simulink model "threeDiskOscillatorRig"  (R2024b)
settings: Solver=VariableStepAuto  StartTime=0.0  StopTime=simTime  RelTol=1e-8
values from neighbouring files (symbols this model uses):
  atan_scale = 100    [threeDiskOscillator.m]
  b_1 = mean(ECP_values([6 7]))    [threeDiskOscillator.m]
  b_2 = mean(ECP_values([8 9]))    [threeDiskOscillator.m]
  b_3 = mean(ECP_values([10 11]))    [threeDiskOscillator.m]
  B_change = [1 0;0 0]    [threeDiskOscillator.m]
  C = [  1 0 0 0 0 0 ... (first row only)    [threeDiskOscillator.m]
  C_aug = [C zeros(3,1)]    [threeDiskOscillator.m]
  C_D = C    [threeDiskOscillator.m]
  C_ref = pinv(C(3,:)/(eye(6) - F_d + G_d*K_c)*G_d*K_c)    [threeDiskOscillator.m]
  C_V_d = C_aug-P_V_d*C_f_aug    [threeDiskOscillator.m]
  F_aug = [F_d G_d(:,1);zeros(1,6) 1]    [threeDiskOscillator.m]
  F_D = F_d - G_f*M_d_va    [threeDiskOscillator.m]
  f_m = [0;0;0]    [threeDiskOscillator.m]
  f_m_time = 8.5    [threeDiskOscillator.m]
  f_u = [0;-0.1]    [threeDiskOscillator.m]
  f_u_time = 25    [threeDiskOscillator.m]
  F_V = F_a-L_V_d*C_f_aug    [threeDiskOscillator.m]
  G_aug = [G_d;0 0]    [threeDiskOscillator.m]
  G_D = G_d - G_f*N_D_d    [threeDiskOscillator.m]
  G_r1u2 = -(1/J_2)*G    [threeDiskOscillator.m]
  G_r1u2_d = c2d(G_r1u2,T_s, 'tustin')    [threeDiskOscillator.m]
  G_r1y1 = -(k_1/J_2)*G    [threeDiskOscillator.m]
  G_r1y1_d = c2d(G_r1y1,T_s, 'tustin')    [threeDiskOscillator.m]
  G_r1y2 = (s^2 + b_2/J_2*s + (k_1+k_2)/J_2)*G    [threeDiskOscillator.m]
  G_r1y2_d = c2d(G_r1y2,T_s, 'tustin')    [threeDiskOscillator.m]
  G_r1y3 = -(k_2/J_2)*G    [threeDiskOscillator.m]
  G_r1y3_d = c2d(G_r1y3,T_s, 'tustin')    [threeDiskOscillator.m]
  G_r2y2 = -(k_2/J_3)*G    [threeDiskOscillator.m]
  G_r2y2_d = c2d(G_r2y2,T_s, 'tustin')    [threeDiskOscillator.m]
  G_r2y3 = (s^2 + b_3/J_3*s + (k_2)/J_3)*G    [threeDiskOscillator.m]
  G_r2y3_d = c2d(G_r2y3,T_s, 'tustin')    [threeDiskOscillator.m]
  G_V = G_a    [threeDiskOscillator.m]
  h = double(vpasolve(eq_1,gg))    [threeDiskOscillator.m]
  J_1 = ECP_values(1)    [threeDiskOscillator.m]
  J_2 = ECP_values(2)    [threeDiskOscillator.m]
  J_3 = ECP_values(3)    [threeDiskOscillator.m]
  k_1 = ECP_values(4)    [threeDiskOscillator.m]
  k_2 = ECP_values(5)    [threeDiskOscillator.m]
  K_c = dlqr(F_d,G_d,Q_c,R_c)    [threeDiskOscillator.m]
  L_aug = dlqe(F_aug,eye(7),C_aug,1e-3*eye(7),sigma_meas(1,1).^2*eye(3))    [threeDiskOscillator.m]
  L_V_d = place(F_a',C_f_aug',vs_eig_d)'    [threeDiskOscillator.m]
  M_d_va = place(F_d,G_f,va_eig_d)    [threeDiskOscillator.m]
  mu_0 = -6.2064e-07    [threeDiskOscillator.m]
  N_D_d = pinv(G_f)*G_f    [threeDiskOscillator.m]
  P_V_d = C_aug*pinv(C_f_aug)    [threeDiskOscillator.m]
  sigma_meas = 0.0093*eye(3)    [threeDiskOscillator.m]
  sigma_r2 = 3.6238e-05    [threeDiskOscillator.m]
  T_Cm = ECP_values(13)    [threeDiskOscillator.m]
  T_Cp = ECP_values(12)    [threeDiskOscillator.m]
  T_s = 0.004    [threeDiskOscillator.m]
  u_fault = 1    [threeDiskOscillator.m]
  w_th = 0.75    [threeDiskOscillator.m]
  x_0 = [0;0;0;0;0;0]    [threeDiskOscillator.m]
undefined symbols (not defined in the file or in its folder): dspblkCoreblockFVToolHelper, gcbh, M
libraries: simulink x1
settings Model: Creator=dimpa  LastModifiedBy=emma
settings SolverCC: AlgebraicLoopSolver=TrustRegion
settings DataIOCC: ReturnWorkspaceOutputs=off
settings DebuggingCC: UnconnectedInputMsg=warning  UnconnectedOutputMsg=warning  UnconnectedLineMsg=warning  ArithmeticOperatorsInVariantConditions=warning
settings ModelReferenceCC: EnableRefExpFcnMdlSchedulingChecks=on
settings SFSimCC: SimUseLocalCustomCode=off  CustomCodeUndefinedFunction=UseInterfaceOnly
settings RTWCC: RTWUseLocalCustomCode=off  GPUComputeCapability=3.5  DLArmComputeVersion=19.05

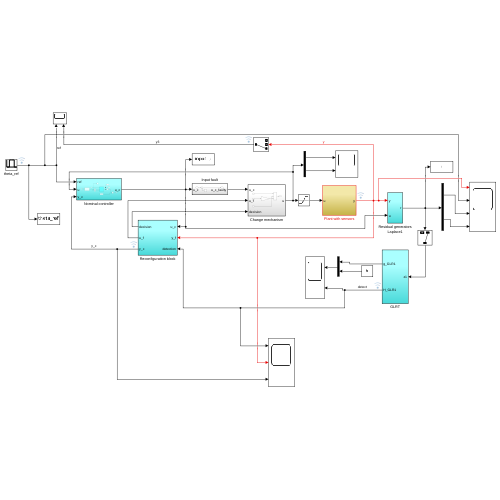
[thumbnail: Simulink's stored preview of the top-level diagram]
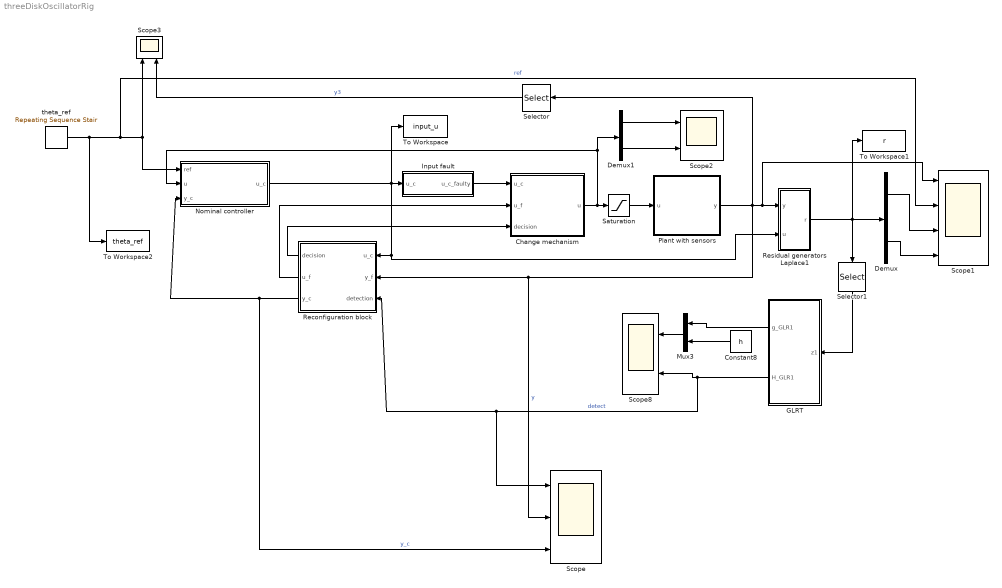
== system threeDiskOscillatorRig ==
  Change mechanism : Subsystem
  Constant8 : Constant  Value=h
  Demux : Demux  Outputs=2
  Demux1 : Demux  Outputs=2
  GLRT : Subsystem
  Input fault : Subsystem
  Mux3 : Mux  Inputs=2
  Nominal controller : Subsystem
  Plant with sensors : Subsystem
  Reconfiguration block : Subsystem
  Residual generators Laplace1 : Subsystem
  Saturation : Saturate  UpperLimit=2  LowerLimit=-2
  Scope : Scope  NumInputPorts=3
  Scope1 : Scope  NumInputPorts=4
  Scope2 : Scope  NumInputPorts=2
  Scope3 : Scope  NumInputPorts=2
  Scope8 : Scope  NumInputPorts=2
  Selector : Selector  InputPortWidth=3  IndexOptions=Index vector (dialog)  Indices=[3]  OutputSizes=1
  Selector1 : Selector  InputPortWidth=2  IndexOptions=Index vector (dialog)  Indices=[2]  OutputSizes=1
  To Workspace : ToWorkspace  VariableName=input_u  SaveFormat=Timeseries  SampleTime=T_s
  To Workspace1 : ToWorkspace  VariableName=r  SaveFormat=Timeseries  SampleTime=T_s
  To Workspace2 : ToWorkspace  VariableName=theta_ref  SaveFormat=Timeseries  SampleTime=T_s
  theta_ref : simulink/Sources/Repeating Sequence Stair  OutValues=[0 1.57 1.57 0]  tsamp=2.5  OutMin=[]  OutMax=[]  OutDataTypeStr=double  OutputDataTypeScalingMode=double  OutDataType=fixdt(0,8)  ConRadixGroup=Best Precision: Vector-wise  OutScaling=2^-12
  wires:
  Selector/1 -> Scope3/2  "y3"
  Saturation/1 -> Plant with sensors/1(u)
  theta_ref/1 -> Scope1/2, Nominal controller/1(ref), Scope3/1, To Workspace2/1  "ref"
  Plant with sensors/1(y) -> Selector/1, Scope/2, Reconfiguration block/2(y_f), Residual generators Laplace1/1(y), Scope1/1  "y"
  Residual generators Laplace1/1(r) -> Selector1/1, Demux/1, To Workspace1/1
  Constant8/1 -> Mux3/2
  Mux3/1 -> Scope8/1
  Demux/1 -> Scope1/3
  Demux/2 -> Scope1/4
  Demux1/1 -> Scope2/1
  Demux1/2 -> Scope2/2
  Nominal controller/1(u_c) -> Input fault/1(u_c), Residual generators Laplace1/2(u), Reconfiguration block/1(u_c), To Workspace/1
  Change mechanism/1(u) -> Nominal controller/2(u), Demux1/1, Saturation/1
  Input fault/1(u_c_faulty) -> Change mechanism/1(u_c)
  Reconfiguration block/1(decision) -> Change mechanism/3(decision)
  Reconfiguration block/2(u_f) -> Change mechanism/2(u_f)
  GLRT/2(H_GLR1) -> Scope/1, Reconfiguration block/3(detection), Scope8/2  "detect"
  GLRT/1(g_GLR1) -> Mux3/1
  Selector1/1 -> GLRT/1(z1)
  Reconfiguration block/3(y_c) -> Scope/3, Nominal controller/3(y_c)  "y_c"

== system threeDiskOscillatorRig/Change mechanism ==
  u_c : Inport
  u_f : Inport  Port=2
  decision : Inport  Port=3
  Gain2 : Gain  Gain=B_change  Multiplication=Matrix(K*u) (u vector)
  Switch2 : Switch  OutDataTypeStr=double  SaturateOnIntegerOverflow=off  InputSameDT=off
  u : Outport
  wires:
  Gain2/1 -> Switch2/3
  decision/1 -> Switch2/2
  u_c/1 -> Switch2/1
  Switch2/1 -> u/1
  u_f/1 -> Gain2/1

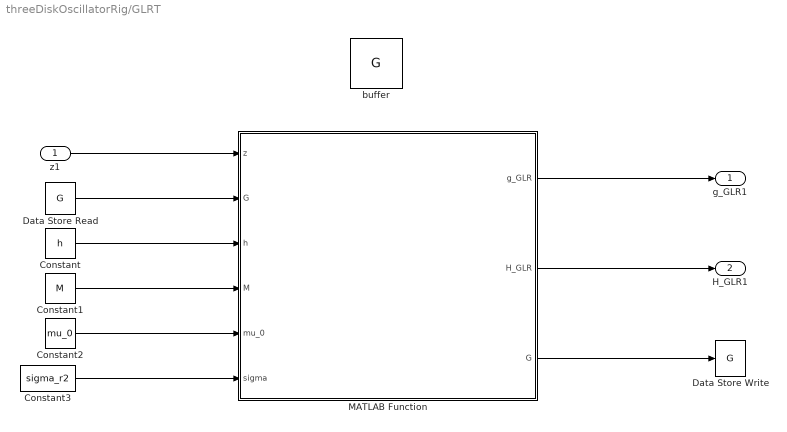
== system threeDiskOscillatorRig/GLRT ==
  z1 : Inport
  Constant : Constant  Value=h
  Constant1 : Constant  Value=M
  Constant2 : Constant  Value=mu_0
  Constant3 : Constant  Value=sigma_r2
  Data Store Read : DataStoreRead  DataStoreName=G  IndexOptions=Index vector (dialog)  Indices=1  OutputSizes=1
  Data Store Write : DataStoreWrite  DataStoreName=G  IndexOptions=Index vector (dialog)  Indices=1  OutputSizes=1
  MATLAB Function : MATLAB Function  TreatAsAtomicUnit=on
  buffer : DataStoreMemory  DataStoreName=G  WriteAfterWriteMsg=warning  InitialValue=zeros(M,1)  ShowAdditionalParam=off
  g_GLR1 : Outport  VectorParamsAs1DForOutWhenUnconnected=off
  H_GLR1 : Outport  Port=2  VectorParamsAs1DForOutWhenUnconnected=off
  wires:
  Constant2/1 -> MATLAB Function/5(mu_0)
  Constant/1 -> MATLAB Function/3(h)
  MATLAB Function/3(G) -> Data Store Write/1
  MATLAB Function/2(H_GLR) -> H_GLR1/1
  Constant1/1 -> MATLAB Function/4(M)
  Data Store Read/1 -> MATLAB Function/2("G ")
  Constant3/1 -> MATLAB Function/6(sigma)
  MATLAB Function/1(g_GLR) -> g_GLR1/1
  z1/1 -> MATLAB Function/1(z)

== system threeDiskOscillatorRig/Input fault ==
  u_c : Inport
  Sum4 : Sum  Inputs=|++
  f_u : Step  Time=f_u_time  After=f_u  SampleTime=0
  u_c_faulty : Outport
  wires:
  f_u/1 -> Sum4/2
  u_c/1 -> Sum4/1
  Sum4/1 -> u_c_faulty/1

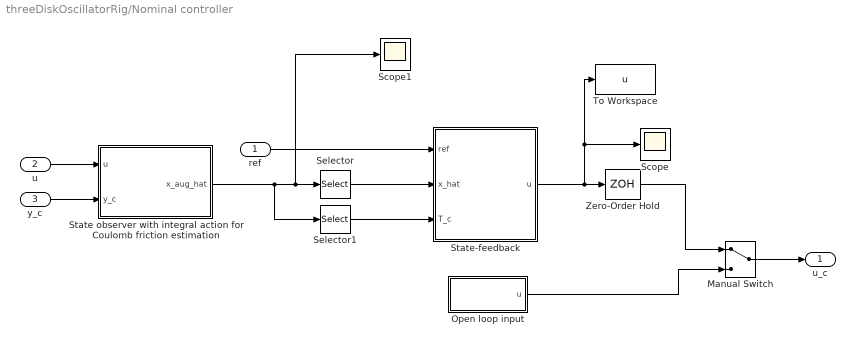
== system threeDiskOscillatorRig/Nominal controller ==
  ref : Inport
  u : Inport  Port=2
  y_c : Inport  Port=3
  Manual Switch : ManualSwitch
  Open loop input : Subsystem
  Scope : Scope
  Scope1 : Scope
  Selector : Selector  InputPortWidth=7  IndexOptions=Index vector (dialog)  Indices=[1:6]  OutputSizes=1
  Selector1 : Selector  InputPortWidth=7  IndexOptions=Index vector (dialog)  Indices=[7]  OutputSizes=1
  State observer with integral action for Coulomb friction estimation : Subsystem
  State-feedback : Subsystem
  To Workspace : ToWorkspace  VariableName=u  SaveFormat=Timeseries  SampleTime=T_s
  Zero-Order Hold : ZeroOrderHold  SampleTime=T_s
  u_c : Outport
  wires:
  Zero-Order Hold/1 -> Manual Switch/1
  y_c/1 -> State observer with integral action for Coulomb friction estimation/2(y_c)
  u/1 -> State observer with integral action for Coulomb friction estimation/1(u)
  Open loop input/1(u) -> Manual Switch/2
  Manual Switch/1 -> u_c/1
  Selector1/1 -> State-feedback/3(T_c)
  State observer with integral action for Coulomb friction estimation/1(x_aug_hat) -> Scope1/1, Selector/1, Selector1/1
  ref/1 -> State-feedback/1(ref)
  State-feedback/1(u) -> To Workspace/1, Scope/1, Zero-Order Hold/1
  Selector/1 -> State-feedback/2(x_hat)

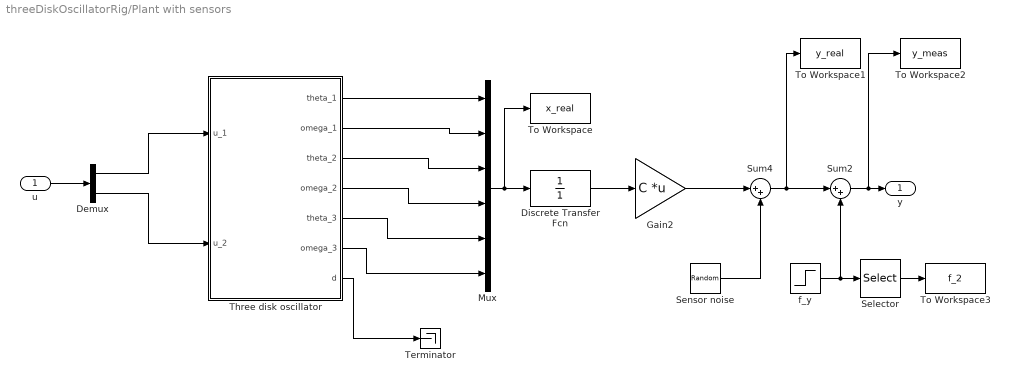
== system threeDiskOscillatorRig/Plant with sensors ==
  u : Inport
  Demux : Demux  Outputs=2
  Discrete Transfer Fcn : DiscreteTransferFcn  LoadFcn=dspblkCoreblockFVToolHelper(gcbh,'load');  Denominator=[1]  SampleTime=T_s
      settings: CopyFcn=dspblkCoreblockFVToolHelper(gcbh,'copy');  DeleteFcn=dspblkCoreblockFVToolHelper(gcbh,'close');  ModelCloseFcn=dspblkCoreblockFVToolHelper(gcbh,'close');  PreSaveFcn=dspblkCoreblockFVToolHelper(gcbh,'presave');  PostSaveFcn=dspblkCoreblockFVToolHelper(gcbh,'postsave');  CloseFcn=dspblkCoreblockFVToolHelper(gcbh,'close');
  Gain2 : Gain  Gain=C  Multiplication=Matrix(K*u) (u vector)
  Mux : Mux  Inputs=6
  Selector : Selector  InputPortWidth=3  IndexOptions=Index vector (dialog)  Indices=[2]  OutputSizes=1
  Sensor noise : RandomNumber  Mean=zeros(3,1)  Variance=diag(sigma_meas^2)  SampleTime=T_s
  Sum2 : Sum  Inputs=|++
  Sum4 : Sum  Inputs=|++
  Terminator : Terminator
  Three disk oscillator : Subsystem
  To Workspace : ToWorkspace  VariableName=x_real  SaveFormat=Timeseries  SampleTime=T_s
  To Workspace1 : ToWorkspace  VariableName=y_real  SaveFormat=Timeseries  SampleTime=T_s
  To Workspace2 : ToWorkspace  VariableName=y_meas  SaveFormat=Timeseries  SampleTime=T_s
  To Workspace3 : ToWorkspace  VariableName=f_2  SaveFormat=Timeseries  SampleTime=T_s
  f_y : Step  Time=f_m_time  Before=[0;0;0]  After=f_m  SampleTime=0
  y : Outport  VectorParamsAs1DForOutWhenUnconnected=off
  wires:
  u/1 -> Demux/1
  Three disk oscillator/2(omega_1) -> Mux/2
  Three disk oscillator/1(theta_1) -> Mux/1
  Mux/1 -> To Workspace/1, Discrete Transfer Fcn/1
  Three disk oscillator/4(omega_2) -> Mux/4
  Three disk oscillator/3(theta_2) -> Mux/3
  Discrete Transfer Fcn/1 -> Gain2/1
  Gain2/1 -> Sum4/1
  Sum4/1 -> To Workspace1/1, Sum2/1
  Sensor noise/1 -> Sum4/2
  Three disk oscillator/6(omega_3) -> Mux/6
  Three disk oscillator/5(theta_3) -> Mux/5
  f_y/1 -> Sum2/2, Selector/1
  Sum2/1 -> To Workspace2/1, y/1
  Selector/1 -> To Workspace3/1
  Demux/1 -> Three disk oscillator/1(u_1)
  Demux/2 -> Three disk oscillator/2(u_2)
  Three disk oscillator/7(d) -> Terminator/1

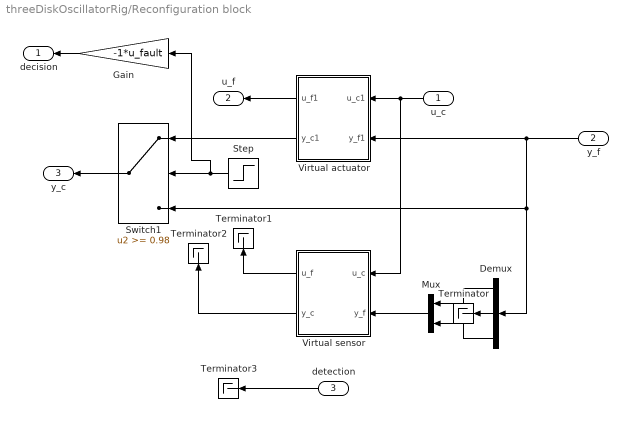
== system threeDiskOscillatorRig/Reconfiguration block ==
  u_c : Inport
  y_f : Inport  Port=2
  detection : Inport  Port=3
  Demux : Demux  Outputs=3
  Gain : Gain  Gain=-1*u_fault
  Mux : Mux  Inputs=2
  Step : Step  Time=f_u_time  SampleTime=0
  Switch1 : Switch  Threshold=0.98  SaturateOnIntegerOverflow=off  InputSameDT=off
  Terminator{,1..3} (4 alike) : Terminator
  Virtual actuator : Subsystem
  Virtual sensor : Subsystem
  decision : Outport  VectorParamsAs1DForOutWhenUnconnected=off
  u_f : Outport  Port=2  VectorParamsAs1DForOutWhenUnconnected=off
  y_c : Outport  Port=3  VectorParamsAs1DForOutWhenUnconnected=off
  wires:
  u_c/1 -> Virtual actuator/1(u_c1), Virtual sensor/1(u_c)
  Switch1/1 -> y_c/1
  Gain/1 -> decision/1
  Virtual sensor/1(u_f) -> Terminator1/1
  Virtual sensor/2(y_c) -> Terminator2/1
  y_f/1 -> Virtual actuator/2(y_f1), Switch1/3, Demux/1
  Demux/1 -> Mux/1
  Demux/3 -> Mux/2
  Demux/2 -> Terminator/1
  Mux/1 -> Virtual sensor/2(y_f)
  Virtual actuator/2(y_c1) -> Switch1/1
  Virtual actuator/1(u_f1) -> u_f/1
  detection/1 -> Terminator3/1
  Step/1 -> Gain/1, Switch1/2

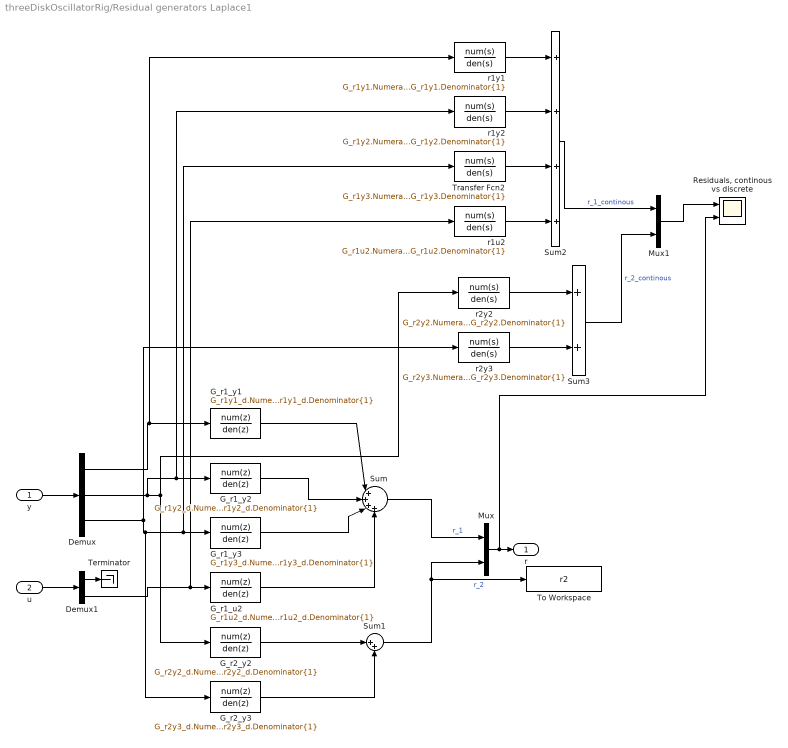
== system threeDiskOscillatorRig/Residual generators Laplace1 ==
  y : Inport
  u : Inport  Port=2
  Demux : Demux  Outputs=3
  Demux1 : Demux  Outputs=2
  G_r1_u2 : DiscreteTransferFcn  Numerator=G_r1u2_d.Numerator{1}  Denominator=G_r1u2_d.Denominator{1}
  G_r1_y1 : DiscreteTransferFcn  Numerator=G_r1y1_d.Numerator{1}  Denominator=G_r1y1_d.Denominator{1}
  G_r1_y2 : DiscreteTransferFcn  Numerator=G_r1y2_d.Numerator{1}  Denominator=G_r1y2_d.Denominator{1}
  G_r1_y3 : DiscreteTransferFcn  Numerator=G_r1y3_d.Numerator{1}  Denominator=G_r1y3_d.Denominator{1}
  G_r2_y2 : DiscreteTransferFcn  LoadFcn=dspblkCoreblockFVToolHelper(gcbh,'load');  Numerator=G_r2y2_d.Numerator{1}  Denominator=G_r2y2_d.Denominator{1}
      settings: CopyFcn=dspblkCoreblockFVToolHelper(gcbh,'copy');  DeleteFcn=dspblkCoreblockFVToolHelper(gcbh,'close');  ModelCloseFcn=dspblkCoreblockFVToolHelper(gcbh,'close');  PreSaveFcn=dspblkCoreblockFVToolHelper(gcbh,'presave');  PostSaveFcn=dspblkCoreblockFVToolHelper(gcbh,'postsave');  CloseFcn=dspblkCoreblockFVToolHelper(gcbh,'close');
  G_r2_y3 : DiscreteTransferFcn  Numerator=G_r2y3_d.Numerator{1}  Denominator=G_r2y3_d.Denominator{1}
  Mux : Mux  Inputs=2
  Mux1 : Mux  Inputs=2
  "Residuals, continous vs discrete" : Scope  NumInputPorts=2
  Sum : Sum  Inputs=|++++
  Sum1 : Sum  Inputs=|++
  Sum2 : Sum  Inputs=++++
  Sum3 : Sum
  Terminator : Terminator
  To Workspace : ToWorkspace  VariableName=r2  SaveFormat=Timeseries  SampleTime=-1
  Transfer Fcn2 : TransferFcn  Numerator=G_r1y3.Numerator{1}  Denominator=G_r1y3.Denominator{1}
  r1u2 : TransferFcn  Numerator=G_r1u2.Numerator{1}  Denominator=G_r1u2.Denominator{1}
  r1y1 : TransferFcn  Numerator=G_r1y1.Numerator{1}  Denominator=G_r1y1.Denominator{1}
  r1y2 : TransferFcn  Numerator=G_r1y2.Numerator{1}  Denominator=G_r1y2.Denominator{1}
  r2y2 : TransferFcn  Numerator=G_r2y2.Numerator{1}  Denominator=G_r2y2.Denominator{1}
  r2y3 : TransferFcn  Numerator=G_r2y3.Numerator{1}  Denominator=G_r2y3.Denominator{1}
  r : Outport  VectorParamsAs1DForOutWhenUnconnected=off
  wires:
  Mux1/1 -> "Residuals, continous vs discrete"/1
  Sum2/1 -> Mux1/1  "r_1_continous"
  Sum3/1 -> Mux1/2  "r_2_continous"
  Demux/2 -> G_r1_y2/1, r1y2/1, G_r2_y2/1, r2y2/1
  r2y2/1 -> Sum3/1
  r2y3/1 -> Sum3/2
  Demux1/1 -> Terminator/1
  r1u2/1 -> Sum2/4
  r1y1/1 -> Sum2/1
  r1y2/1 -> Sum2/2
  Transfer Fcn2/1 -> Sum2/3
  Demux/3 -> r2y3/1, G_r1_y3/1, Transfer Fcn2/1, G_r2_y3/1
  G_r1_u2/1 -> Sum/4
  G_r1_y3/1 -> Sum/3
  G_r1_y2/1 -> Sum/2
  G_r2_y3/1 -> Sum1/2
  G_r2_y2/1 -> Sum1/1
  Demux1/2 -> G_r1_u2/1, r1u2/1
  G_r1_y1/1 -> Sum/1
  Demux/1 -> G_r1_y1/1, r1y1/1
  Sum1/1 -> To Workspace/1, Mux/2  "r_2"
  Sum/1 -> Mux/1  "r_1"
  u/1 -> Demux1/1
  Mux/1 -> r/1, "Residuals, continous vs discrete"/2
  y/1 -> Demux/1

== system threeDiskOscillatorRig/Nominal controller/Open loop input ==
  Constant : Constant  Value=3
  Constant1 : Constant  Value=0
  Multiport Switch : MultiPortSwitch  SaturateOnIntegerOverflow=off  InputSameDT=off
  Mux : Mux  Inputs=2
  Mux1 : Mux  Inputs=2
  Mux2 : Mux  Inputs=2
  Pulse Generator : DiscretePulseGenerator  PulseType=Time based  Period=10  PulseWidth=5
  u : Outport
  wires:
  Constant1/1 -> Mux1/1, Mux/2
  Pulse Generator/1 -> Mux2/2, Mux2/1, Mux1/2, Mux/1
  Constant/1 -> Multiport Switch/1
  Mux2/1 -> Multiport Switch/4
  Mux/1 -> Multiport Switch/2
  Multiport Switch/1 -> u/1
  Mux1/1 -> Multiport Switch/3

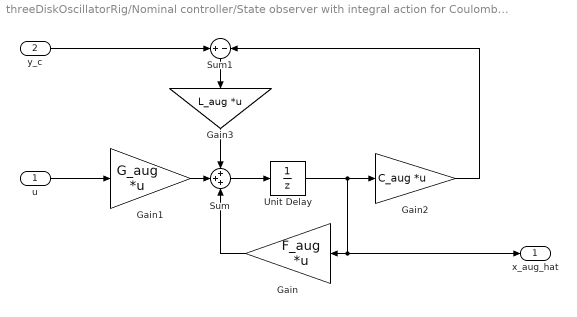
== system threeDiskOscillatorRig/Nominal controller/State observer with integral action for Coulomb friction estimation ==
  u : Inport
  y_c : Inport  Port=2
  Gain : Gain  Gain=F_aug  Multiplication=Matrix(K*u) (u vector)
  Gain1 : Gain  Gain=G_aug  Multiplication=Matrix(K*u) (u vector)
  Gain2 : Gain  Gain=C_aug  Multiplication=Matrix(K*u) (u vector)
  Gain3 : Gain  Gain=L_aug  Multiplication=Matrix(K*u) (u vector)
  Sum : Sum  Inputs=+++
  Sum1 : Sum  Inputs=+-
  Unit Delay : UnitDelay  SampleTime=T_s  HasFrameUpgradeWarning=on
  x_aug_hat : Outport  VectorParamsAs1DForOutWhenUnconnected=off
  wires:
  Unit Delay/1 -> x_aug_hat/1, Gain/1, Gain2/1
  y_c/1 -> Sum1/1
  Sum1/1 -> Gain3/1
  Sum/1 -> Unit Delay/1
  Gain2/1 -> Sum1/2
  u/1 -> Gain1/1
  Gain1/1 -> Sum/2
  Gain/1 -> Sum/3
  Gain3/1 -> Sum/1

== system threeDiskOscillatorRig/Nominal controller/State-feedback ==
  note: Feed-forward term for Coulomb friction
  ref : Inport
  x_hat : Inport  Port=2
  T_c : Inport  Port=3
  Gain2 : Gain  Gain=[1;0]
  State feedback controller : Subsystem
  Sum2 : Sum  Inputs=|+-
  u : Outport  VectorParamsAs1DForOutWhenUnconnected=off
  wires:
  T_c/1 -> Gain2/1
  Gain2/1 -> Sum2/2
  Sum2/1 -> u/1
  ref/1 -> State feedback controller/1(ref)
  x_hat/1 -> State feedback controller/2(x_hat)
  State feedback controller/1(u_fb) -> Sum2/1

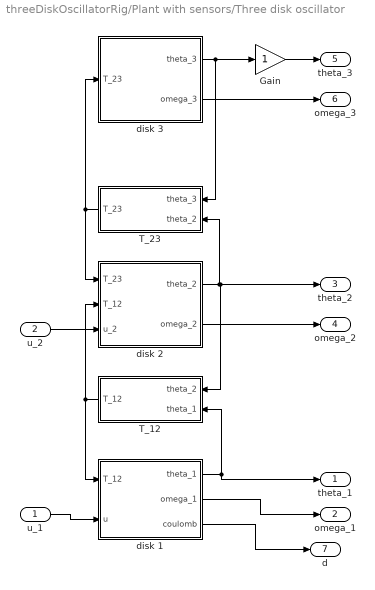
== system threeDiskOscillatorRig/Plant with sensors/Three disk oscillator ==
  u_1 : Inport
  u_2 : Inport  Port=2
  Gain : Gain
  T_12 : Subsystem
  T_23 : Subsystem
  disk 1 : Subsystem
  disk 2 : Subsystem
  disk 3 : Subsystem
  theta_1 : Outport  VectorParamsAs1DForOutWhenUnconnected=off
  omega_1 : Outport  Port=2  VectorParamsAs1DForOutWhenUnconnected=off
  theta_2 : Outport  Port=3  VectorParamsAs1DForOutWhenUnconnected=off
  omega_2 : Outport  Port=4  VectorParamsAs1DForOutWhenUnconnected=off
  theta_3 : Outport  Port=5  VectorParamsAs1DForOutWhenUnconnected=off
  omega_3 : Outport  Port=6  VectorParamsAs1DForOutWhenUnconnected=off
  d : Outport  Port=7  VectorParamsAs1DForOutWhenUnconnected=off
  wires:
  T_23/1(T_23) -> disk 2/1(T_23), disk 3/1(T_23)
  disk 1/1(theta_1) -> theta_1/1, T_12/2(theta_1)
  disk 2/1(theta_2) -> T_23/2(theta_2), theta_2/1, T_12/1(theta_2)
  T_12/1(T_12) -> disk 1/1(T_12), disk 2/2(T_12)
  disk 3/2(omega_3) -> omega_3/1
  disk 1/2(omega_1) -> omega_1/1
  disk 2/2(omega_2) -> omega_2/1
  u_1/1 -> disk 1/2(u)
  disk 3/1(theta_3) -> Gain/1, T_23/1(theta_3)
  Gain/1 -> theta_3/1
  u_2/1 -> disk 2/3(u_2)
  disk 1/3(coulomb) -> d/1

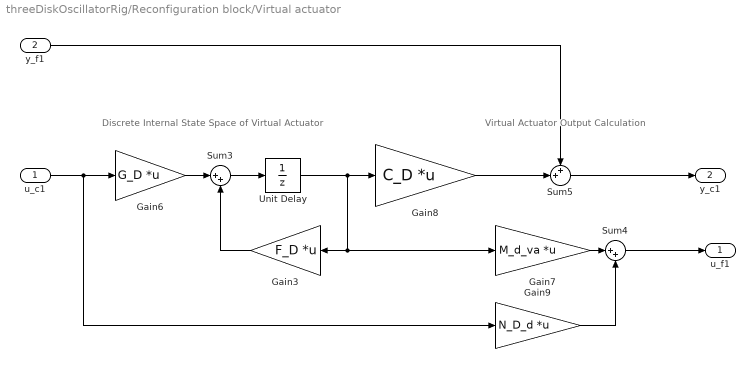
== system threeDiskOscillatorRig/Reconfiguration block/Virtual actuator ==
  note: Virtual Actuator Output Calculation
  note: Discrete Internal State Space of Virtual Actuator
  u_c1 : Inport
  y_f1 : Inport  Port=2
  Gain3 : Gain  Gain=F_D  Multiplication=Matrix(K*u) (u vector)
  Gain6 : Gain  Gain=G_D  Multiplication=Matrix(K*u) (u vector)
  Gain7 : Gain  Gain=M_d_va  Multiplication=Matrix(K*u) (u vector)
  Gain8 : Gain  Gain=C_D  Multiplication=Matrix(K*u) (u vector)
  Gain9 : Gain  Gain=N_D_d  Multiplication=Matrix(K*u) (u vector)
  Sum3 : Sum  Inputs=|++
  Sum4 : Sum  Inputs=|++
  Sum5 : Sum  Inputs=++|
  Unit Delay : UnitDelay  SampleTime=-1  HasFrameUpgradeWarning=on
  u_f1 : Outport  VectorParamsAs1DForOutWhenUnconnected=off
  y_c1 : Outport  Port=2  VectorParamsAs1DForOutWhenUnconnected=off
  wires:
  Sum3/1 -> Unit Delay/1
  Gain7/1 -> Sum4/1
  Unit Delay/1 -> Gain7/1, Gain3/1, Gain8/1
  Gain9/1 -> Sum4/2
  Sum4/1 -> u_f1/1
  Gain6/1 -> Sum3/1
  Gain8/1 -> Sum5/2
  Sum5/1 -> y_c1/1
  y_f1/1 -> Sum5/1
  Gain3/1 -> Sum3/2
  u_c1/1 -> Gain9/1, Gain6/1

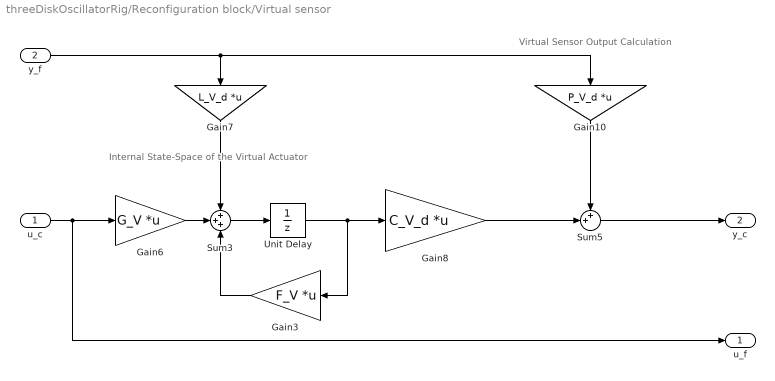
== system threeDiskOscillatorRig/Reconfiguration block/Virtual sensor ==
  note: Virtual Sensor Output Calculation
  note: Internal State-Space of the Virtual Actuator
  u_c : Inport
  y_f : Inport  Port=2
  Gain10 : Gain  Gain=P_V_d  Multiplication=Matrix(K*u) (u vector)
  Gain3 : Gain  Gain=F_V  Multiplication=Matrix(K*u) (u vector)
  Gain6 : Gain  Gain=G_V  Multiplication=Matrix(K*u) (u vector)
  Gain7 : Gain  Gain=L_V_d  Multiplication=Matrix(K*u) (u vector)
  Gain8 : Gain  Gain=C_V_d  Multiplication=Matrix(K*u) (u vector)
  Sum3 : Sum  Inputs=+++
  Sum5 : Sum  Inputs=++|
  Unit Delay : UnitDelay  SampleTime=-1  HasFrameUpgradeWarning=on
  u_f : Outport  VectorParamsAs1DForOutWhenUnconnected=off
  y_c : Outport  Port=2  VectorParamsAs1DForOutWhenUnconnected=off
  wires:
  Gain7/1 -> Sum3/1
  Gain3/1 -> Sum3/3
  Gain8/1 -> Sum5/2
  Sum5/1 -> y_c/1
  Gain6/1 -> Sum3/2
  y_f/1 -> Gain10/1, Gain7/1
  u_c/1 -> u_f/1, Gain6/1
  Gain10/1 -> Sum5/1
  Sum3/1 -> Unit Delay/1
  Unit Delay/1 -> Gain3/1, Gain8/1

== system threeDiskOscillatorRig/Nominal controller/State-feedback/State feedback controller ==
  ref : Inport
  x_hat : Inport  Port=2
  Gain5 : Gain  Gain=C_ref  Multiplication=Matrix(K*u) (u vector)
  Gain6 : Gain  Gain=K_c  Multiplication=Matrix(K*u) (u vector)
  Scope1 : Scope  NumInputPorts=2
  Sum2 : Sum  Inputs=|+-
  u_fb : Outport
  wires:
  Gain5/1 -> Sum2/1
  x_hat/1 -> Sum2/2
  ref/1 -> Gain5/1
  Sum2/1 -> Gain6/1
  Gain6/1 -> u_fb/1

== system threeDiskOscillatorRig/Plant with sensors/Three disk oscillator/T_12 ==
  theta_2 : Inport
  theta_1 : Inport  Port=2
  Gain : Gain  Gain=k_1
  Sum : Sum  Inputs=|+-
  T_12 : Outport  VectorParamsAs1DForOutWhenUnconnected=off
  wires:
  theta_2/1 -> Sum/2
  theta_1/1 -> Sum/1
  Sum/1 -> Gain/1
  Gain/1 -> T_12/1

== system threeDiskOscillatorRig/Plant with sensors/Three disk oscillator/T_23 ==
  theta_3 : Inport
  theta_2 : Inport  Port=2
  Gain : Gain  Gain=k_2
  Sum : Sum  Inputs=-+|
  T_23 : Outport  VectorParamsAs1DForOutWhenUnconnected=off
  wires:
  Gain/1 -> T_23/1
  Sum/1 -> Gain/1
  theta_3/1 -> Sum/1
  theta_2/1 -> Sum/2

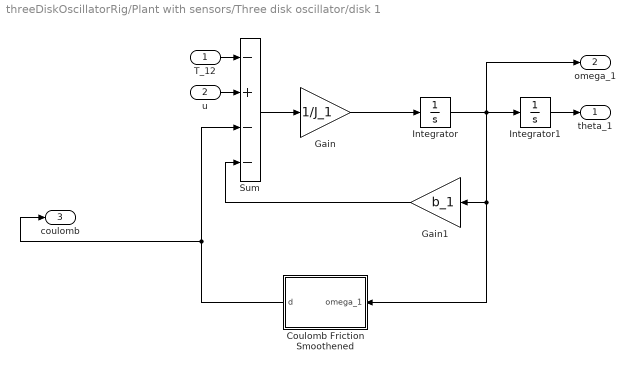
== system threeDiskOscillatorRig/Plant with sensors/Three disk oscillator/disk 1 ==
  T_12 : Inport
  u : Inport  Port=2
  Coulomb Friction Smoothened : Subsystem
  Gain : Gain  Gain=1/J_1
  Gain1 : Gain  Gain=b_1
  Integrator : Integrator  InitialCondition=x_0(2)
  Integrator1 : Integrator  InitialCondition=x_0(1)
  Sum : Sum  Inputs=-+--
  theta_1 : Outport  VectorParamsAs1DForOutWhenUnconnected=off
  omega_1 : Outport  Port=2  VectorParamsAs1DForOutWhenUnconnected=off
  coulomb : Outport  Port=3  VectorParamsAs1DForOutWhenUnconnected=off
  wires:
  Sum/1 -> Gain/1
  Integrator/1 -> Integrator1/1, omega_1/1, Coulomb Friction Smoothened/1(omega_1), Gain1/1
  Gain1/1 -> Sum/4
  Integrator1/1 -> theta_1/1
  T_12/1 -> Sum/1
  u/1 -> Sum/2
  Gain/1 -> Integrator/1
  Coulomb Friction Smoothened/1(d) -> coulomb/1, Sum/3

== system threeDiskOscillatorRig/Plant with sensors/Three disk oscillator/disk 2 ==
  T_23 : Inport
  T_12 : Inport  Port=2
  u_2 : Inport  Port=3
  Gain : Gain  Gain=1/J_2
  Gain1 : Gain  Gain=b_2
  Integrator : Integrator  InitialCondition=x_0(4)
  Integrator1 : Integrator  InitialCondition=x_0(3)
  Sum : Sum  Inputs=+-+-
  theta_2 : Outport  VectorParamsAs1DForOutWhenUnconnected=off
  omega_2 : Outport  Port=2  VectorParamsAs1DForOutWhenUnconnected=off
  wires:
  T_23/1 -> Sum/2
  T_12/1 -> Sum/1
  Integrator1/1 -> theta_2/1
  Gain1/1 -> Sum/4
  Gain/1 -> Integrator/1
  Integrator/1 -> Integrator1/1, Gain1/1, omega_2/1
  Sum/1 -> Gain/1
  u_2/1 -> Sum/3

== system threeDiskOscillatorRig/Plant with sensors/Three disk oscillator/disk 3 ==
  T_23 : Inport
  Gain : Gain  Gain=1/J_3
  Gain1 : Gain  Gain=b_3
  Integrator : Integrator  InitialCondition=x_0(6)
  Integrator1 : Integrator  InitialCondition=x_0(5)
  Sum : Sum  Inputs=|+-
  theta_3 : Outport  VectorParamsAs1DForOutWhenUnconnected=off
  omega_3 : Outport  Port=2  VectorParamsAs1DForOutWhenUnconnected=off
  wires:
  Sum/1 -> Gain/1
  Integrator/1 -> Integrator1/1, omega_3/1, Gain1/1
  Gain/1 -> Integrator/1
  Gain1/1 -> Sum/2
  Integrator1/1 -> theta_3/1
  T_23/1 -> Sum/1

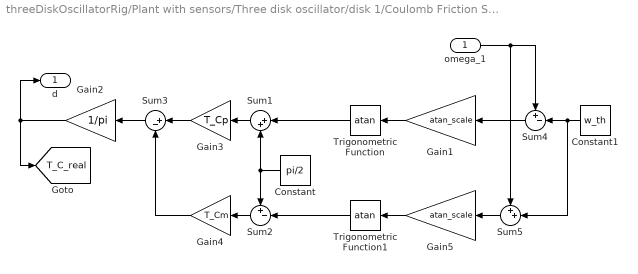
== system threeDiskOscillatorRig/Plant with sensors/Three disk oscillator/disk 1/Coulomb Friction Smoothened ==
  omega_1 : Inport
  Constant : Constant  Value=pi/2
  Constant1 : Constant  Value=w_th
  Gain1 : Gain  Gain=atan_scale
  Gain2 : Gain  Gain=1/pi
  Gain3 : Gain  Gain=T_Cp
  Gain4 : Gain  Gain=T_Cm
  Gain5 : Gain  Gain=atan_scale
  Sum1 : Sum  Inputs=|++
  Sum2 : Sum  Inputs=+-|
  Sum3 : Sum  Inputs=|+-
  Sum4 : Sum  Inputs=+-|
  Sum5 : Sum  Inputs=++|
  Trigonometric Function : Trigonometry  Operator=atan
  Trigonometric Function1 : Trigonometry  Operator=atan
  d : Outport  VectorParamsAs1DForOutWhenUnconnected=off
  tag scope: T_C_real=global
  wires:
  Gain1/1 -> Trigonometric Function/1
  Sum1/1 -> Gain3/1
  Constant/1 -> Sum2/1, Sum1/2
  Sum2/1 -> Gain4/1
  Sum3/1 -> Gain2/1
  Trigonometric Function/1 -> Sum1/1
  Gain4/1 -> Sum3/2
  Gain2/1 -> [T_C_real], d/1
  omega_1/1 -> Sum5/1, Sum4/1
  Gain3/1 -> Sum3/1
  Sum4/1 -> Gain1/1
  Constant1/1 -> Sum5/2, Sum4/2
  Gain5/1 -> Trigonometric Function1/1
  Sum5/1 -> Gain5/1
  Trigonometric Function1/1 -> Sum2/2

== matlab function threeDiskOscillatorRig/GLRT/MATLAB Function ==
  data: z input; g_GLR output; H_GLR output; G input; G output; h input; M input; mu_0 input; sigma input
function [g_GLR, H_GLR, G] = GLR(z, G, h, M, mu_0, sigma)

G = [G(2:end); z];
maxi = 0;
for i = 1:M
    s = sum(G(M-i+1:end) - mu_0);
    tmp = (s^2) / i;
    if tmp > maxi
        maxi = tmp;
    end
end

g_GLR = maxi/(2*sigma);
H_GLR = (g_GLR>h);
